simulink model "test_lift_motion_law_no_ctrl"  (R2021b)
settings: Solver=VariableStepAuto  StartTime=0.0  StopTime=150  RelTol=1e-3
values from neighbouring files (symbols this model uses):
  gearbox = 1    [load_data.m]    (also in run_test_motion_law_block.m; run_test_motion_logic.m; test_motion_law.m)
  Rp = 0.5    [load_data.m]    (also in run_test_motion_law_block.m; run_test_motion_logic.m; test_motion_law.m)
  Ts = 1e-3    (= 0.001)    [load_data.m]    (also in run_test_motion_law_block.m; run_test_motion_logic.m; run_test_switch_sensor.m; testWegMotionLaw.m)
libraries: LiftMotionControlLibrary x4
settings Model: Creator=manue  LastModifiedBy=manue
settings ConfigComp: PLC_TargetIDE=generic  PLC_MultiTBSigbuilderTimeRange=off  PLC_InlineEnumCastFunction=off

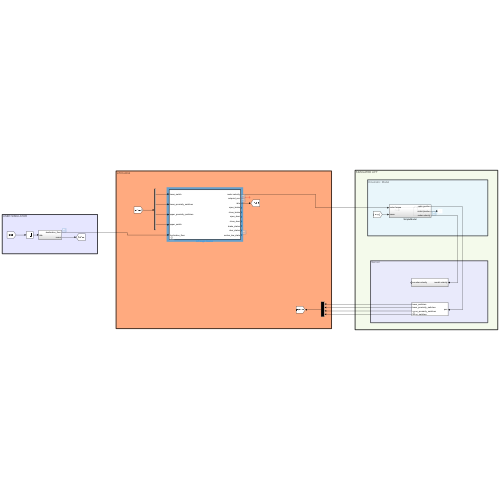
[thumbnail: Simulink's stored preview of the top-level diagram]
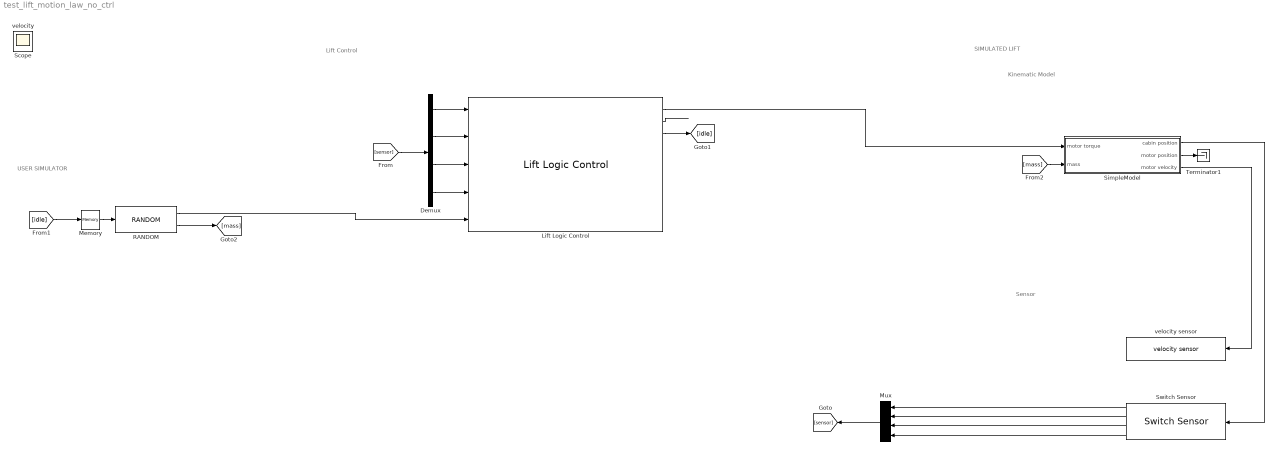
== system test_lift_motion_law_no_ctrl ==
  note: SIMULATED LIFT
  note: USER SIMULATOR
  note: Sensor
  note: Kinematic Model
  note: Lift Control
  Demux : Demux
  Lift Logic Control : LiftMotionControlLibrary/Lift Logic Control  num_floors=num_floors  Ts=Ts  gearbox=gearbox  Rp=Rp  waiting_time_open_door=waiting_time_open_door  waiting_time_close_door=waiting_time_close_door  waiting_time_open_brake=waiting_time_open_brake  waiting_time_close_brake_copy=waiting_time_close_brake  waiting_time_steady_state=waiting_time_steady_state  HighSpeed=HighSpeed  LowSpeed=LowSpeed  PercentAccFactor=PercentAccFactor  AccelInitialJerk=AccelInitialJerk  Acceleration=Acceleration  AccelEndJerk=AccelEndJerk  DecelInitialJerk=DecelInitialJerk  Deceleration=Deceleration  DecelEndJerk=DecelEndJerk  StopDeceleration=StopDeceleration
  Memory : Memory
  Mux : Mux
  RANDOM : LiftMotionControlLibrary/RANDOM  SystemSampleTime=-1  VariantActivationTime=update diagram  Latency=0  AutoFrameSizeCalculation=off
  SimpleModel : Subsystem
  Switch Sensor : LiftMotionControlLibrary/Switch Sensor  lower_proximity_sensor_positions=lower_proximity_sensor_positions  upper_proximity_sensor_positions=upper_proximity_sensor_positions  lower_floor_sensor_positions=lower_floor_sensor_positions  upper_floor_sensor_positions=upper_floor_sensor_positions  num_floors=num_floors  sensor_height=sensor_height
  Terminator1 : Terminator
  velocity sensor : LiftMotionControlLibrary/velocity sensor  SystemSampleTime=-1  VariantActivationTime=update diagram  Latency=0  AutoFrameSizeCalculation=off
  Scope : Scope
  velocity : Scope
  wires:
  Switch Sensor/1 -> Mux/1
  Switch Sensor/2 -> Mux/2
  Switch Sensor/3 -> Mux/3
  Demux/3 -> Lift Logic Control/3
  Demux/2 -> Lift Logic Control/2
  Demux/1 -> Lift Logic Control/1
  Mux/1 -> [sensor]
  [sensor] -> Demux/1
  SimpleModel/2(motor position) -> Terminator1/1
  Lift Logic Control/1 -> SimpleModel/1(motor torque)
  Lift Logic Control/3 -> [idle]
  RANDOM/2 -> [mass]
  [mass] -> SimpleModel/2(mass)
  [idle] -> Memory/1
  Memory/1 -> RANDOM/1
  SimpleModel/3(motor velocity) -> velocity sensor/1
  SimpleModel/1(cabin position) -> Switch Sensor/1
  RANDOM/1 -> Lift Logic Control/5
  Demux/4 -> Lift Logic Control/4
  Switch Sensor/4 -> Mux/4
  Lift Logic Control/2 -> ?

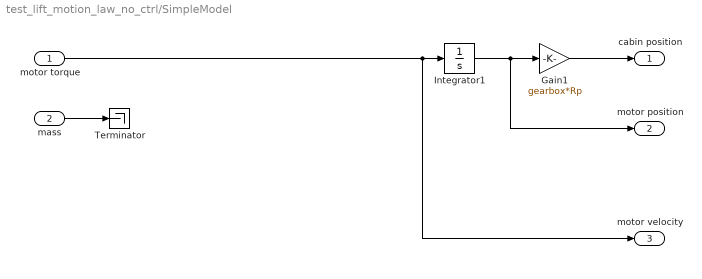
== system test_lift_motion_law_no_ctrl/SimpleModel ==
  motor torque : Inport
  mass : Inport  Port=2
  Gain1 : Gain  Gain=gearbox*Rp
  Integrator1 : Integrator
  Terminator : Terminator
  cabin position : Outport
  motor position : Outport  Port=2
  motor velocity : Outport  Port=3
  wires:
  motor torque/1 -> motor velocity/1, Integrator1/1
  Integrator1/1 -> motor position/1, Gain1/1
  Gain1/1 -> cabin position/1
  mass/1 -> Terminator/1
